simulink model "Question2_1"  (R2020b)
settings: Solver=FixedStepAuto  StartTime=0.0  StopTime=100.0  FixedStep=0.01  RelTol=1e-3
settings Model: Creator=Murat  LastModifiedBy=Murat

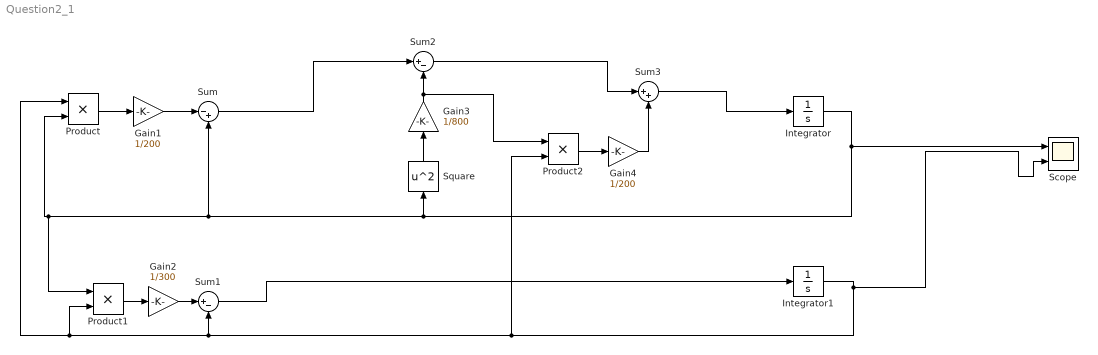
== system Question2_1 ==
  Gain1 : Gain  Gain=1/200
  Gain2 : Gain  Gain=1/300
  Gain3 : Gain  Gain=1/800
  Gain4 : Gain  Gain=1/200
  Integrator : Integrator  InitialCondition=400
  Integrator1 : Integrator  InitialCondition=100
  Product : Product
  Product1 : Product
  Product2 : Product
  Scope : Scope  NumInputPorts=2
  Square : Math  Operator=square  SaturateOnIntegerOverflow=on
  Sum : Sum  Inputs=|-+
  Sum1 : Sum  Inputs=|+-
  Sum2 : Sum  Inputs=|+-
  Sum3 : Sum  Inputs=|++
  wires:
  Sum1/1 -> Integrator1/1
  Integrator/1 -> Scope/1, Square/1, Product1/1, Product/2, Sum/2
  Product/1 -> Gain1/1
  Gain2/1 -> Sum1/1
  Integrator1/1 -> Scope/2, Product2/2, Product/1, Product1/2, Sum1/2
  Product1/1 -> Gain2/1
  Gain1/1 -> Sum/1
  Square/1 -> Gain3/1
  Gain3/1 -> Product2/1, Sum2/2
  Sum/1 -> Sum2/1
  Product2/1 -> Gain4/1
  Sum2/1 -> Sum3/1
  Gain4/1 -> Sum3/2
  Sum3/1 -> Integrator/1
